simulink model "Final_Dual2"  (R2025a)
settings: Solver=ode113  StartTime=0.0  StopTime=1800  FixedStep=0.01  MaxStep=0.1  RelTol=1e-3
undefined symbols (not defined in the file or in its folder): sigbuilder_block
libraries: simulink x3784, slpidlib x2
(part 2 of 161)

== system Final_Dual2/VehicleDynamics//RoadLoadModel ==
  TqAct : Inport
  Veh_Mass : Inport  Port=2
  Road_mu : Inport  Port=3
  Gear_ratio : Inport  Port=4
  Tyre_radius : Inport  Port=5
  2 : Constant  Value=0  SampleTime=-1
  2pi : Constant  Value=2*pi  SampleTime=-1
  3 : Constant  Value=0  SampleTime=-1
  Add4 : Sum
  Constant : Constant
  Constant1 : Constant  Value=2*pi
  Constant2 : Constant  Value=60/1000
  Delay : Delay  DelayLength=1
  Divide{,1..3} (4 alike) : Product  Inputs=*/
  Gain1 : Gain  Gain=-1
  Integrator : Integrator
  Product{1..4} (4 alike) : Product
  Product5 : Product  Inputs=4
  Product9 : Product  Inputs=3
  Rate Transition : RateTransition
  Saturation : Saturate  UpperLimit=30000  LowerLimit=-30000
  Sec2Min : Gain  Gain=60
  Sum : Sum
  Switch1 : Switch  Criteria=u2 > Threshold  Threshold=10  SaturateOnIntegerOverflow=off  InputSameDT=off
  Switch2 : Switch  Criteria=u2 > Threshold  Threshold=-10  SaturateOnIntegerOverflow=off  InputSameDT=off
  TmEta : Gain  Gain=0.96
  g-value : Constant  Value=9.8  SampleTime=-1
  RPM : Outport
  tag scope: Vehicle_Acceleration=global, Vehicle_Speed_kmph=global, rpm_final=global
  wires:
  Road_mu/1 -> Product9/3
  Divide/1 -> Sum/2
  Product3/1 -> Divide1/2
  Tyre_radius/1 -> Product1/2, Product3/2, Divide/2
  Product4/1 -> Divide/1
  Divide2/1 -> [Vehicle_Acceleration], Integrator/1  "Vehicle acceleration"
  Sum/1 -> Divide2/1  "Traction Force"
  Integrator/1 -> Sec2Min/1  "velocity"
  2pi/1 -> Product3/1
  TqAct/1 -> TmEta/1
  Sec2Min/1 -> Divide1/1  "velocity in min"
  Divide1/1 -> Product2/1  "wheelrpm"
  Veh_Mass/1 -> Divide2/2, Product9/1
  g-value/1 -> Product9/2
  Product2/1 -> Saturation/1
  Switch1/1 -> Gain1/1
  2/1 -> Switch1/3
  Product9/1 -> Switch1/1, Switch2/3  "Friction loss"
  [rpm_final] -> Switch1/2, Switch2/2
  Switch2/1 -> Add4/2
  3/1 -> Switch2/1
  Gain1/1 -> Add4/1
  Add4/1 -> Sum/1
  Gear_ratio/1 -> Product4/2, Divide3/2, Product2/2
  TmEta/1 -> Product4/1
  Saturation/1 -> Delay/1, RPM/1  "Motor RPM"
  Delay/1 -> Rate Transition/1
  Rate Transition/1 -> Product5/1, [rpm_final]
  Constant/1 -> Divide3/1
  Constant1/1 -> Product1/1
  Divide3/1 -> Product5/2
  Product1/1 -> Product5/3
  Constant2/1 -> Product5/4
  Product5/1 -> [Vehicle_Speed_kmph]

== system Final_Dual2/WLTP (3) ==
  Demux : Demux  Tag=STV Demux  Outputs=1
      settings: DisplayOption=none
  FromWs : FromWorkspace  Tag=STV FromWs  VariableName=tuvar
      SigBuilderData=|
      | common.afterFinalStr = 'Extrapolate'
      | common.sampleTime = 0
      | dataSet.timeRange = [0 3593]
      | dataSet.name = 'Sheet1'
      | sbobj.Name = 'Signal Builder'
      | sbobj.Groups.Name = 'Sheet1'
      | sbobj.Groups.Signals.Name = 'WLTP'
      | sbobj.Groups.Signals.XData = [0 1 2 3 4 5 6 7 8 9 10 11 ... (3594 elements, 1x3594)]
      | sbobj.Groups.Signals.YData = [0 0 0 0 0 0 0 0 0 0 0 0.06 ... (3594 elements, 1x3594)]
      | sbobj.Groups.TimeRange = [0 3593]
  WLTP : Outport  Tag=STV Outport
  wires:
  Demux/1 -> WLTP/1
  FromWs/1 -> Demux/1

== system Final_Dual2/Battery1/Module1 ==
  Module_Current : Inport
  Add : Sum  Inputs=++++++++++
  Add1 : Sum  Inputs=++++++++++
  Constant : Constant  Value=10
  Divide : Product  Inputs=*/
  Scope : Scope
      settings: DataLoggingSaveFormat=Array
  Scope1 : Scope
      settings: DataLoggingVariableName=ScopeData3  DataLoggingSaveFormat=Array
  SubModule_1 : Subsystem
  SubModule_10 : Subsystem
  SubModule_2 : Subsystem
  SubModule_3 : Subsystem
  SubModule_4 : Subsystem
  SubModule_5 : Subsystem
  SubModule_6 : Subsystem
  SubModule_7 : Subsystem
  SubModule_8 : Subsystem
  SubModule_9 : Subsystem
  Module_Voltage : Outport
  Module_avg_Temp : Outport  Port=2
  wires:
  SubModule_4/2(SubModule_avg_temp) -> Add1/4
  Add/1 -> Module_Voltage/1, Scope/1
  [Module_Current] -> SubModule_5/1(Module_Current)
  [Module_Current] -> SubModule_9/1(Module_Current)
  [Module_Current] -> SubModule_2/1(Module_Current)
  [Module_Current] -> SubModule_3/1(Module_Current)
  [Module_Current] -> SubModule_7/1(Module_Current)
  Module_Current/1 -> [Module_Current]
  SubModule_1/1(SubModule_Voltage) -> Add/1
  [Module_Current] -> SubModule_1/1(Module_Current)
  [Module_Current] -> SubModule_4/1(Module_Current)
  SubModule_6/2(SubModule_avg_temp) -> Add1/6
  Divide/1 -> Module_avg_Temp/1, Scope1/1
  SubModule_5/1(SubModule_Voltage) -> Add/5
  [Module_Current] -> SubModule_8/1(Module_Current)
  SubModule_8/2(SubModule_avg_temp) -> Add1/8
  SubModule_5/2(SubModule_avg_temp) -> Add1/5
  SubModule_8/1(SubModule_Voltage) -> Add/8
  [Module_Current] -> SubModule_10/1(Module_Current)
  Constant/1 -> Divide/2
  SubModule_10/1(SubModule_Voltage) -> Add/10
  SubModule_10/2(SubModule_avg_temp) -> Add1/10
  SubModule_7/1(SubModule_Voltage) -> Add/7
  SubModule_9/2(SubModule_avg_temp) -> Add1/9
  SubModule_3/1(SubModule_Voltage) -> Add/3
  SubModule_4/1(SubModule_Voltage) -> Add/4
  SubModule_2/2(SubModule_avg_temp) -> Add1/2
  SubModule_3/2(SubModule_avg_temp) -> Add1/3
  SubModule_7/2(SubModule_avg_temp) -> Add1/7
  Add1/1 -> Divide/1
  SubModule_9/1(SubModule_Voltage) -> Add/9
  SubModule_6/1(SubModule_Voltage) -> Add/6
  SubModule_2/1(SubModule_Voltage) -> Add/2
  SubModule_1/2(SubModule_avg_temp) -> Add1/1
  [Module_Current] -> SubModule_6/1(Module_Current)

== system Final_Dual2/Battery1/Module2 ==
  Module_Current : Inport
  Add : Sum  Inputs=++++++++++
  Add1 : Sum  Inputs=++++++++++
  Constant : Constant  Value=10
  Divide : Product  Inputs=*/
  Scope : Scope
      settings: DataLoggingSaveFormat=Array
  Scope1 : Scope
      settings: DataLoggingVariableName=ScopeData3  DataLoggingSaveFormat=Array
  SubModule_1 : Subsystem
  SubModule_10 : Subsystem
  SubModule_2 : Subsystem
  SubModule_3 : Subsystem
  SubModule_4 : Subsystem
  SubModule_5 : Subsystem
  SubModule_6 : Subsystem
  SubModule_7 : Subsystem
  SubModule_8 : Subsystem
  SubModule_9 : Subsystem
  Module_Voltage : Outport
  Module_avg_Temp : Outport  Port=2
  wires:
  SubModule_4/2(SubModule_avg_temp) -> Add1/4
  Add/1 -> Module_Voltage/1, Scope/1
  [Module_Current] -> SubModule_5/1(Module_Current)
  [Module_Current] -> SubModule_9/1(Module_Current)
  [Module_Current] -> SubModule_2/1(Module_Current)
  [Module_Current] -> SubModule_3/1(Module_Current)
  [Module_Current] -> SubModule_7/1(Module_Current)
  Module_Current/1 -> [Module_Current]
  SubModule_1/1(SubModule_Voltage) -> Add/1
  [Module_Current] -> SubModule_1/1(Module_Current)
  [Module_Current] -> SubModule_4/1(Module_Current)
  SubModule_6/2(SubModule_avg_temp) -> Add1/6
  Divide/1 -> Module_avg_Temp/1, Scope1/1
  SubModule_5/1(SubModule_Voltage) -> Add/5
  [Module_Current] -> SubModule_8/1(Module_Current)
  SubModule_8/2(SubModule_avg_temp) -> Add1/8
  SubModule_5/2(SubModule_avg_temp) -> Add1/5
  SubModule_8/1(SubModule_Voltage) -> Add/8
  [Module_Current] -> SubModule_10/1(Module_Current)
  Constant/1 -> Divide/2
  SubModule_10/1(SubModule_Voltage) -> Add/10
  SubModule_10/2(SubModule_avg_temp) -> Add1/10
  SubModule_7/1(SubModule_Voltage) -> Add/7
  SubModule_9/2(SubModule_avg_temp) -> Add1/9
  SubModule_3/1(SubModule_Voltage) -> Add/3
  SubModule_4/1(SubModule_Voltage) -> Add/4
  SubModule_2/2(SubModule_avg_temp) -> Add1/2
  SubModule_3/2(SubModule_avg_temp) -> Add1/3
  SubModule_7/2(SubModule_avg_temp) -> Add1/7
  Add1/1 -> Divide/1
  SubModule_9/1(SubModule_Voltage) -> Add/9
  SubModule_6/1(SubModule_Voltage) -> Add/6
  SubModule_2/1(SubModule_Voltage) -> Add/2
  SubModule_1/2(SubModule_avg_temp) -> Add1/1
  [Module_Current] -> SubModule_6/1(Module_Current)

== system Final_Dual2/Battery1/Module3 ==
  Module_Current : Inport
  Add : Sum  Inputs=++++++++++
  Add1 : Sum  Inputs=++++++++++
  Constant : Constant  Value=10
  Divide : Product  Inputs=*/
  Scope : Scope
      settings: DataLoggingSaveFormat=Array
  Scope1 : Scope
      settings: DataLoggingVariableName=ScopeData3  DataLoggingSaveFormat=Array
  SubModule_1 : Subsystem
  SubModule_10 : Subsystem
  SubModule_2 : Subsystem
  SubModule_3 : Subsystem
  SubModule_4 : Subsystem
  SubModule_5 : Subsystem
  SubModule_6 : Subsystem
  SubModule_7 : Subsystem
  SubModule_8 : Subsystem
  SubModule_9 : Subsystem
  Module_Voltage : Outport
  Module_avg_Temp : Outport  Port=2
  wires:
  [Module_Current] -> SubModule_6/1(Module_Current)
  SubModule_1/2(SubModule_avg_temp) -> Add1/1
  SubModule_2/1(SubModule_Voltage) -> Add/2
  SubModule_6/1(SubModule_Voltage) -> Add/6
  SubModule_9/1(SubModule_Voltage) -> Add/9
  Add1/1 -> Divide/1
  SubModule_7/2(SubModule_avg_temp) -> Add1/7
  SubModule_3/2(SubModule_avg_temp) -> Add1/3
  SubModule_2/2(SubModule_avg_temp) -> Add1/2
  SubModule_4/1(SubModule_Voltage) -> Add/4
  SubModule_3/1(SubModule_Voltage) -> Add/3
  SubModule_9/2(SubModule_avg_temp) -> Add1/9
  SubModule_7/1(SubModule_Voltage) -> Add/7
  SubModule_10/2(SubModule_avg_temp) -> Add1/10
  SubModule_10/1(SubModule_Voltage) -> Add/10
  Constant/1 -> Divide/2
  [Module_Current] -> SubModule_10/1(Module_Current)
  SubModule_8/1(SubModule_Voltage) -> Add/8
  SubModule_5/2(SubModule_avg_temp) -> Add1/5
  SubModule_8/2(SubModule_avg_temp) -> Add1/8
  [Module_Current] -> SubModule_8/1(Module_Current)
  SubModule_5/1(SubModule_Voltage) -> Add/5
  Divide/1 -> Scope1/1, Module_avg_Temp/1
  SubModule_6/2(SubModule_avg_temp) -> Add1/6
  [Module_Current] -> SubModule_4/1(Module_Current)
  [Module_Current] -> SubModule_1/1(Module_Current)
  SubModule_1/1(SubModule_Voltage) -> Add/1
  Module_Current/1 -> [Module_Current]
  [Module_Current] -> SubModule_7/1(Module_Current)
  [Module_Current] -> SubModule_3/1(Module_Current)
  [Module_Current] -> SubModule_2/1(Module_Current)
  [Module_Current] -> SubModule_9/1(Module_Current)
  [Module_Current] -> SubModule_5/1(Module_Current)
  Add/1 -> Scope/1, Module_Voltage/1
  SubModule_4/2(SubModule_avg_temp) -> Add1/4

== system Final_Dual2/Battery1/NMC_Cell_Config ==
  A : Constant  Value=0.013
  C1_User1 : Constant  Value=[800 850 900 950 1000 1050 1000 950 900 850 800]
  C2_User : Constant  Value=[15 16 17 18 19 20 19 18 17 16 15]
  Cell_Capacity_Ah_rated : Constant  Value=26.5
  Gain1 : Gain  Gain=1e-03
  Gain2 : Gain
  Gain3 : Gain  Gain=1e-03
  Gain4 : Gain  Gain=1e+03
  Gain5 : Gain  Gain=0.01
  Gain6 : Gain  Gain=1e-04
  Goto11 : Goto  TagVisibility=global
  M*Cp : Constant  Value=369
  OCV_NMC : Constant  Value=|
      | [
      |     2.954364, 3.109857, 3.273534, 3.3066, 3.34,    3.3734,  3.20473;
      |     3.122427, 3.286765, 3.459753, 3.4947, 3.53,    3.5653,  3.387035;
      |     3.175499, 3.342631, 3.518559, 3.5541, 3.59,    3.6259,  3.444605;
      |     3.210881, 3.379875, 3.557763, 3.5937, 3.63,    3.6663,  3.482985;
      |     3.237417, 3.407808, 3.587166, 3.6234, 3.66,    3.6966,  3.511777;
      |     3.272799, 3.445052, 3.62637,  3.663,  3.7,     3.737,   3.55015;
      |     3.317026, 3.491066, 3.675375, 3.7125, 3.75,    3.7875,  3.598125;
      |     3.387789, 3.566094, 3.753783, 3.7917, 3.83,    3.8683,  3.674885;
      |     3.467398, 3.649892, 3.841992, 3.8808, 3.92,    3.9592,  3.76124;
      |     3.564697, 3.752313, 3.949803, 3.9897, 4.03,    4.0703,  3.866785;
      |     3.653151, 3.845422, 4.047813, 4.0887, 4.13,    4.1713,  3.962735
      | ]
  R1_User : Constant  Value=[1.5 1.2 0.9 0.7 0.6 0.5 0.5 0.5 0.6 0.7 0.8]
  R2_User1 : Constant  Value=[2.5 2 1.6 1.3 1.1 1 1.1 1.2 1.3 1.4 1.5]
  Ri_NMC : Constant  Value=|
      | [67.2155, 61.105, 55.55, 55, 52.25, 49.6375, 54.60125;
      |     48.884, 44.44, 40.4, 40, 38, 36.1, 39.71;
      |     44.60665, 40.5515, 36.865, 36.5, 34.675, 32.94125, 36.23538;
      |     41.5514, 37.774, 34.34, 34, 32.83, 30.685, 33.7535;
      |     40.3293, 36.663, 33.33, 33, 31.35, 29.7825, 32.76075;
      |     39.71825, 36.1075, 32.825, 32.5, 31.25, 29.33125, 32.26438;
      |     40.08488, 36.4408, 33.128, 32.8, 31.16, 29.602, 32.5622;
      |     40.94035, 37.2185, 33.835, 33.5, 31.825, 30.23375, 33.15738;
      |     42.7735, 38.1925, 35.03, 34.7, 32.375, 31.5875, 34.74263;
      |     51.3282, 46.602, 42.42, 42, 39.9, 37.905, 41.6955;
      |     73.326, 66.66, 60.6, 60, 57, 54.15, 59.565]
  SOC_Initial_% : Constant  Value=100
  SOC_User : Constant  Value=[0 10 20 30 40 50 60 70 80 90 100]
  Temp_Initial_degC : Constant  Value=25
  Temp_ambient : Constant  Value=25
  h : Constant  Value=20
  tag scope: C1_User=global, C2_User=global, Cell_Capacity=global, Cp=global, OCV=global, R1_User=global, R2_User=global, Ri_User=global, SOC_Iinitial=global, SOC_User=global, Temp_Iinitial=global, Temp_ambient=global, h=global
  wires:
  OCV_NMC/1 -> [OCV]
  SOC_User/1 -> Gain5/1
  R1_User/1 -> Gain1/1
  Gain1/1 -> [R1_User]
  C1_User1/1 -> Gain2/1
  Gain2/1 -> [C1_User]
  R2_User1/1 -> Gain3/1
  Gain3/1 -> [R2_User]
  Gain4/1 -> [C2_User]
  C2_User/1 -> Gain4/1
  Cell_Capacity_Ah_rated/1 -> [Cell_Capacity]
  SOC_Initial_%/1 -> [SOC_Iinitial]
  Gain5/1 -> [SOC_User]
  Temp_Initial_degC/1 -> [Temp_ambient], [Temp_Iinitial]
  h/1 -> [h]
  A/1 -> Goto11/1
  M*Cp/1 -> [Cp]
  Gain6/1 -> [Ri_User]
  Ri_NMC/1 -> Gain6/1

== system Final_Dual2/Battery1/SOCEstimator ==
  SOC_Initial : Inport
  Pack_Capacity : Inport  Port=2
  Current : Inport  Port=3
  SOCEstimator : Subsystem
  SOC : Outport
  wires:
  SOCEstimator/1(SOC) -> SOC/1
  SOC_Initial/1 -> SOCEstimator/1(SOC_Initial)
  Current/1 -> SOCEstimator/2(Current)
  Pack_Capacity/1 -> SOCEstimator/3(CellCapacity)

== system Final_Dual2/Battery2/LTO_Cell_Config ==
  A : Constant  Value=0.0344
  C1_User1 : Constant  Value=[5.0, 9.0, 12.0, 14.0, 14.8, 15.0, 14.8, 13.0, 10.0, 7.0, 4.5]
  C2_User : Constant  Value=[50, 90, 130, 160, 168, 170, 168, 155, 120, 80, 45]
  Cell_Capacity_Ah_rated : Constant  Value=23
  Gain1 : Gain  Gain=1e-03
  Gain2 : Gain  Gain=1e+03
  Gain3 : Gain  Gain=1e-03
  Gain4 : Gain  Gain=1e+03
  Gain5 : Gain  Gain=0.01
  Gain6 : Gain  Gain=1e-03
  M*Cp : Constant  Value=632.5
  OCV_LTO : Constant  Value=|
      | [1.79,  1.77,   1.76,   1.74,   1.71,   1.69,   1.66;
      |     2.09,  2.09,   2.08,   2.07,   2.06,   2.05,   2.04;
      |     2.19,  2.19,   2.18,   2.18,   2.17,   2.16,   2.15;
      |     2.23,  2.23,   2.23,   2.22,   2.22,   2.21,   2.21;
      |     2.25,  2.25,   2.25,   2.24,   2.24,   2.23,   2.23;
      |     2.28,  2.27,   2.27,   2.27,   2.26,   2.26,   2.25;
      |     2.30,  2.29,   2.29,   2.29,   2.28,   2.28,   2.27;
      |     2.32,  2.31,   2.31,   2.31,   2.30,   2.30,   2.29;
      |     2.34,  2.34,   2.34,   2.33,   2.33,   2.32,   2.31;
      |     2.39,  2.39,   2.38,   2.38,   2.37,   2.36,   2.35;
      |     2.64,  2.62,   2.61,   2.60,   2.59,   2.58,   2.57]
  R1_User : Constant  Value=[1.00, 0.65, 0.50, 0.40, 0.37, 0.35, 0.37, 0.45, 0.60, 0.80, 1.10]
  R2_User1 : Constant  Value=[2.00, 1.20, 0.90, 0.70, 0.62, 0.60, 0.62, 0.75, 1.00, 1.50, 2.20]
  Ri_LTO : Constant  Value=[2.50,1.90,1.65,1.50,1.40,1.30,1.25;1.50,1.10,0.90,0.80,0.75,0.72,0.70;1.25,0.95,0.75,0.65,0.60,0.58,0.57;1.10,0.80,0.60,0.52,0.48,0.47,0.46;1.05,0.75,0.55,0.48,0.45,0.44,0.43;1.00,0.70,0.52,0.45,0.42,0.41,0.40;1.05,0.75,0.55,0.48,0.45,0.44,0.43;1.15,0.85,0.65,0.57,0.53,0.51,0.50;1.40,1.05,0.85,0.75,0.70,0.68,0.67;1.80,1.40,1.15,1.00,0.90,0.85,0.82;2.20,1.70,1.40,1.25,1.15,1.10,1.05]
  SOC_Initial_% : Constant  Value=100
  SOC_User : Constant  Value=[0 10 20 30 40 50 60 70 80 90 100]
  Temp_Initial_degC : Constant  Value=25
  h : Constant  Value=25
  tag scope: A_LTO=global, C1_User_LTO=global, C2_User_LTO=global, Cell_Capacity_LTO=global, Cp_LTO=global, OCV_LTO=global, R1_User_LTO=global, R2_User_LTO=global, Ri_User_LTO=global, SOC_Iinitial_LTO=global, SOC_User_LTO=global, Temp_Iinitial_LTO=global, h_LTO=global
  wires:
  OCV_LTO/1 -> [OCV_LTO]
  SOC_User/1 -> Gain5/1
  R1_User/1 -> Gain1/1
  Gain1/1 -> [R1_User_LTO]
  C1_User1/1 -> Gain2/1
  Gain2/1 -> [C1_User_LTO]
  R2_User1/1 -> Gain3/1
  Gain3/1 -> [R2_User_LTO]
  Gain4/1 -> [C2_User_LTO]
  C2_User/1 -> Gain4/1
  Cell_Capacity_Ah_rated/1 -> [Cell_Capacity_LTO]
  SOC_Initial_%/1 -> [SOC_Iinitial_LTO]
  Gain5/1 -> [SOC_User_LTO]
  Temp_Initial_degC/1 -> [Temp_Iinitial_LTO]
  h/1 -> [h_LTO]
  A/1 -> [A_LTO]
  M*Cp/1 -> [Cp_LTO]
  Gain6/1 -> [Ri_User_LTO]
  Ri_LTO/1 -> Gain6/1

== system Final_Dual2/Battery2/Module1 ==
  Module_Current : Inport
  Add : Sum
  Add1 : Sum
  Constant : Constant  Value=2
  Divide : Product  Inputs=*/
  Scope : Scope
      settings: DataLoggingSaveFormat=Array
  Scope1 : Scope
      settings: ActiveDisplayYMinimum=53.8572  ActiveDisplayYMaximum=77.3331  DataLoggingVariableName=ScopeData3  DataLoggingSaveFormat=Array
  SubModule_1 : Subsystem
  SubModule_2 : Subsystem
  Module_Voltage : Outport
  Module_avg_Temp : Outport  Port=2
  wires:
  Add/1 -> Module_Voltage/1, Scope/1
  Module_Current/1 -> [Module_Current]
  SubModule_1/1(SubModule_Voltage) -> Add/1
  [Module_Current] -> SubModule_1/1(Module_Current)
  Divide/1 -> Module_avg_Temp/1, Scope1/1
  Constant/1 -> Divide/2
  Add1/1 -> Divide/1
  [Module_Current] -> SubModule_2/1(Module_Current)
  SubModule_2/1(SubModule_Voltage) -> Add/2
  SubModule_1/2(SubModule_avg_temp) -> Add1/1
  SubModule_2/2(SubModule_avg_temp) -> Add1/2

== system Final_Dual2/Battery2/Module2 ==
  Module_Current : Inport
  Add : Sum
  Add1 : Sum
  Constant : Constant  Value=2
  Divide : Product  Inputs=*/
  Scope : Scope
      settings: DataLoggingSaveFormat=Array
  Scope1 : Scope
      settings: ActiveDisplayYMinimum=53.8572  ActiveDisplayYMaximum=77.3331  DataLoggingVariableName=ScopeData3  DataLoggingSaveFormat=Array
  SubModule_1 : Subsystem
  SubModule_2 : Subsystem
  Module_Voltage : Outport
  Module_avg_Temp : Outport  Port=2
  wires:
  SubModule_2/2(SubModule_avg_temp) -> Add1/2
  SubModule_1/2(SubModule_avg_temp) -> Add1/1
  SubModule_2/1(SubModule_Voltage) -> Add/2
  [Module_Current] -> SubModule_2/1(Module_Current)
  Add1/1 -> Divide/1
  Constant/1 -> Divide/2
  Divide/1 -> Scope1/1, Module_avg_Temp/1
  [Module_Current] -> SubModule_1/1(Module_Current)
  SubModule_1/1(SubModule_Voltage) -> Add/1
  Module_Current/1 -> [Module_Current]
  Add/1 -> Scope/1, Module_Voltage/1

== system Final_Dual2/Battery2/SOCEstimator ==
  SOC_Initial : Inport
  Pack_Capacity : Inport  Port=2
  Current : Inport  Port=3
  SOCEstimator : Subsystem
  SOC : Outport
  wires:
  SOCEstimator/1(SOC) -> SOC/1
  SOC_Initial/1 -> SOCEstimator/1(SOC_Initial)
  Current/1 -> SOCEstimator/2(Current)
  Pack_Capacity/1 -> SOCEstimator/3(CellCapacity)

== system Final_Dual2/Observations/Battery1 Operation ==
  Battery1_Voltage : Inport
  Battery1_Current : Inport  Port=2
  Battery1_DischargeCurrLim : Inport  Port=3
  Battery1_ChargeCurrLim : Inport  Port=4
  Battery1_SOC : Inport  Port=5
  Battery1_Temperature : Inport  Port=6
  Battery1_Power : Inport  Port=7
  Battery1_Currents,Current_Limits&SOC : Scope  NumInputPorts=2
      settings: ActiveDisplayYMinimum=-203.9141  ActiveDisplayYMaximum=272.28558  DataLoggingVariableName=ScopeData2
  Battery1_Power&Temperature : Scope  NumInputPorts=2
      settings: ActiveDisplayYMinimum=24.76608  ActiveDisplayYMaximum=27.10528  DataLoggingVariableName=ScopeData3
  Battery1_Voltage&SOC : Scope  NumInputPorts=2
      settings: ActiveDisplayYMinimum=749.76765  ActiveDisplayYMaximum=933.2467
  Mux : Mux  Inputs=3
  wires:
  Battery1_Voltage/1 -> Battery1_Voltage&SOC/1
  Battery1_SOC/1 -> Battery1_Voltage&SOC/2, Battery1_Currents,Current_Limits&SOC/2
  Mux/1 -> Battery1_Currents,Current_Limits&SOC/1
  Battery1_Current/1 -> Mux/1
  Battery1_DischargeCurrLim/1 -> Mux/2
  Battery1_ChargeCurrLim/1 -> Mux/3
  Battery1_Temperature/1 -> Battery1_Power&Temperature/1
  Battery1_Power/1 -> Battery1_Power&Temperature/2

== system Final_Dual2/Observations/Battery2 Operation ==
  Battery2_Voltage : Inport
  Battery2_Current : Inport  Port=2
  Battery2_DischargeCurrLim : Inport  Port=3
  Battery2_ChargeCurrLim : Inport  Port=4
  Battery2_SOC : Inport  Port=5
  Battery2_Temperature : Inport  Port=6
  Battery2_Power : Inport  Port=7
  Battery2_Currents,Current_Limits&SOC : Scope  NumInputPorts=2
      settings: ActiveDisplayYMinimum=-965.27695  ActiveDisplayYMaximum=1034.84646  DataLoggingVariableName=ScopeData2
  Battery2_Power&Temperature : Scope  NumInputPorts=2
      settings: DataLoggingVariableName=ScopeData3
  Battery2_Voltage&SOC : Scope  NumInputPorts=2
      settings: ActiveDisplayYMinimum=63.66915  ActiveDisplayYMaximum=145.68331
  Mux : Mux  Inputs=3
  wires:
  Battery2_SOC/1 -> Battery2_Voltage&SOC/2, Battery2_Currents,Current_Limits&SOC/2
  Battery2_Voltage/1 -> Battery2_Voltage&SOC/1
  Battery2_ChargeCurrLim/1 -> Mux/3
  Battery2_Temperature/1 -> Battery2_Power&Temperature/1
  Battery2_Power/1 -> Battery2_Power&Temperature/2
  Battery2_DischargeCurrLim/1 -> Mux/2
  Battery2_Current/1 -> Mux/1
  Mux/1 -> Battery2_Currents,Current_Limits&SOC/1

== system Final_Dual2/Observations/DAB & Load Splitter Operation ==
  DAB_HighSideCurrentRef : Inport
  DAB_HighSideCurrent : Inport  Port=2
  DAB_PowerTransfer : Inport  Port=3
  Battery1_Current : Inport  Port=4
  Battery2_Current : Inport  Port=5
  Total_Current : Inport  Port=6
  Currents : Scope  NumInputPorts=2
      settings: ActiveDisplayYMinimum=-101.22034  ActiveDisplayYMaximum=330.24185  DataLoggingVariableName=ScopeData6
  DAB_HighSideCurr : Scope  NumInputPorts=2
      settings: ActiveDisplayYMinimum=-74.13996  ActiveDisplayYMaximum=160.56624  DataLoggingVariableName=ScopeData4
  DAB_Power : Scope
      settings: ActiveDisplayYMinimum=-56.99649  ActiveDisplayYMaximum=71.85076  DataLoggingVariableName=ScopeData5
  Mux : Mux  Inputs=3
  wires:
  DAB_PowerTransfer/1 -> DAB_Power/1
  DAB_HighSideCurrent/1 -> DAB_HighSideCurr/2, Mux/2
  Battery1_Current/1 -> Mux/1
  Total_Current/1 -> Mux/3
  DAB_HighSideCurrentRef/1 -> DAB_HighSideCurr/1
  Mux/1 -> Currents/1
  Battery2_Current/1 -> Currents/2

== system Final_Dual2/Observations/System Operation ==
  RPM_request : Inport
  RPM_Actual : Inport  Port=2
  Vehicle_Speed : Inport  Port=3
  Electrical_Power : Inport  Port=4
  Mechanical_Power : Inport  Port=5
  System_Efficiency : Inport  Port=6
  Driveline_Torque_Request : Inport  Port=7
  Driveline_Torque : Inport  Port=8
  Motor_Torque : Inport  Port=9
  Vehicle_Acceleration : Inport  Port=10
  Mux : Mux  Inputs=2
  Mux1 : Mux  Inputs=2
  Mux2 : Mux  Inputs=2
  Power&Efficiency : Scope  NumInputPorts=2
      settings: ActiveDisplayYMinimum=-94.56358  ActiveDisplayYMaximum=255.83618  DataLoggingVariableName=ScopeData8
  RPM_Requested&Actual : Scope  NumInputPorts=2
      settings: ActiveDisplayYMinimum=-2187.5  ActiveDisplayYMaximum=19687.5  DataLoggingVariableName=ScopeData7
  Requested&Actual_Torques : Scope  NumInputPorts=2
      settings: ActiveDisplayYMinimum=-861.66528  ActiveDisplayYMaximum=540.18503  DataLoggingVariableName=ScopeData9
  VehicleSpeed&Acceleration : Scope  NumInputPorts=2
      settings: ActiveDisplayYMinimum=-2187.5  ActiveDisplayYMaximum=19687.5  DataLoggingVariableName=ScopeData10
  wires:
  RPM_request/1 -> Mux2/1
  RPM_Actual/1 -> Mux2/2
  Electrical_Power/1 -> Mux/1
  Mechanical_Power/1 -> Mux/2
  System_Efficiency/1 -> Power&Efficiency/2
  Mux/1 -> Power&Efficiency/1
  Mux1/1 -> Requested&Actual_Torques/1
  Driveline_Torque_Request/1 -> Mux1/1
  Driveline_Torque/1 -> Mux1/2
  Motor_Torque/1 -> Requested&Actual_Torques/2
  Vehicle_Speed/1 -> VehicleSpeed&Acceleration/1, RPM_Requested&Actual/2
  Mux2/1 -> RPM_Requested&Actual/1
  Vehicle_Acceleration/1 -> VehicleSpeed&Acceleration/2

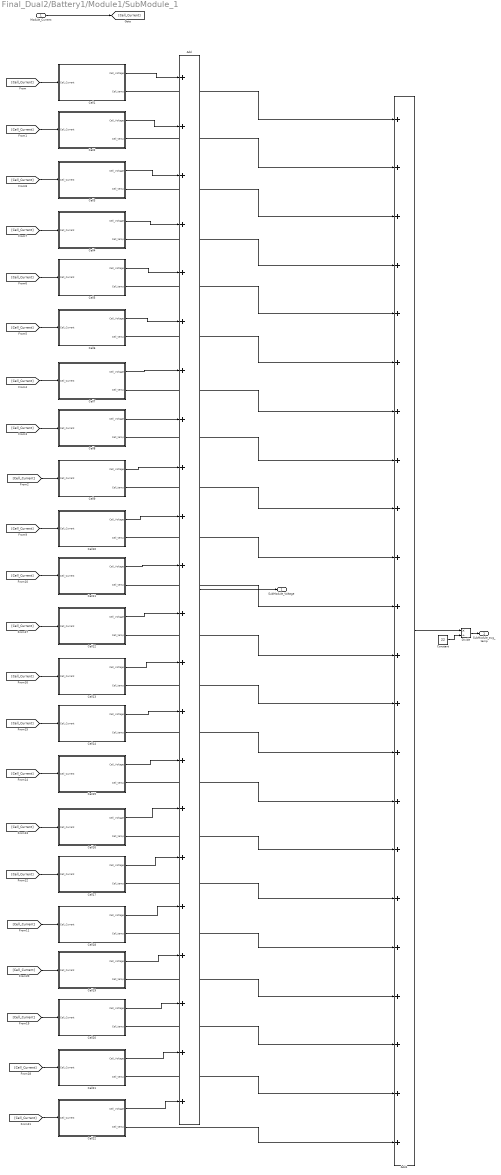
== system Final_Dual2/Battery1/Module1/SubModule_1 ==
  Module_Current : Inport
  Add : Sum  Inputs=++++++++++++++++++++++
  Add1 : Sum  Inputs=++++++++++++++++++++++
  Cell1 : Subsystem
  Cell10 : Subsystem
  Cell11 : Subsystem
  Cell12 : Subsystem
  Cell13 : Subsystem
  Cell14 : Subsystem
  Cell15 : Subsystem
  Cell16 : Subsystem
  Cell17 : Subsystem
  Cell18 : Subsystem
  Cell19 : Subsystem
  Cell2 : Subsystem
  Cell20 : Subsystem
  Cell21 : Subsystem
  Cell22 : Subsystem
  Cell3 : Subsystem
  Cell4 : Subsystem
  Cell5 : Subsystem
  Cell6 : Subsystem
  Cell7 : Subsystem
  Cell8 : Subsystem
  Cell9 : Subsystem
  Constant : Constant  Value=22
  Divide : Product  Inputs=*/
  SubModule_Voltage : Outport
  SubModule_avg_temp : Outport  Port=2
  wires:
  Cell9/2(Cell_temp) -> Add1/9
  [Cell_Current] -> Cell8/1(Cell_Current)
  Cell13/1(Cell_Voltage) -> Add/13
  Cell4/1(Cell_Voltage) -> Add/4
  Module_Current/1 -> [Cell_Current]
  Cell15/1(Cell_Voltage) -> Add/15
  [Cell_Current] -> Cell7/1(Cell_Current)
  [Cell_Current] -> Cell10/1(Cell_Current)
  Cell21/2(Cell_temp) -> Add1/21
  Cell5/1(Cell_Voltage) -> Add/5
  [Cell_Current] -> Cell1/1(Cell_Current)
  Cell2/1(Cell_Voltage) -> Add/2
  Cell19/1(Cell_Voltage) -> Add/19
  [Cell_Current] -> Cell5/1(Cell_Current)
  [Cell_Current] -> Cell11/1(Cell_Current)
  Cell6/1(Cell_Voltage) -> Add/6
  Cell11/1(Cell_Voltage) -> Add/11
  [Cell_Current] -> Cell18/1(Cell_Current)
  Cell7/2(Cell_temp) -> Add1/7
  [Cell_Current] -> Cell21/1(Cell_Current)
  [Cell_Current] -> Cell12/1(Cell_Current)
  [Cell_Current] -> Cell4/1(Cell_Current)
  Cell18/1(Cell_Voltage) -> Add/18
  Cell20/1(Cell_Voltage) -> Add/20
  Cell11/2(Cell_temp) -> Add1/11
  [Cell_Current] -> Cell2/1(Cell_Current)
  Cell16/2(Cell_temp) -> Add1/16
  [Cell_Current] -> Cell15/1(Cell_Current)
  [Cell_Current] -> Cell6/1(Cell_Current)
  [Cell_Current] -> Cell13/1(Cell_Current)
  Cell2/2(Cell_temp) -> Add1/2
  Cell22/2(Cell_temp) -> Add1/22
  Cell9/1(Cell_Voltage) -> Add/9
  Cell7/1(Cell_Voltage) -> Add/7
  [Cell_Current] -> Cell9/1(Cell_Current)
  Cell14/2(Cell_temp) -> Add1/14
  Cell17/1(Cell_Voltage) -> Add/17
  Cell10/2(Cell_temp) -> Add1/10
  [Cell_Current] -> Cell16/1(Cell_Current)
  Cell8/1(Cell_Voltage) -> Add/8
  Cell21/1(Cell_Voltage) -> Add/21
  Cell12/2(Cell_temp) -> Add1/12
  Cell22/1(Cell_Voltage) -> Add/22
  [Cell_Current] -> Cell20/1(Cell_Current)
  [Cell_Current] -> Cell17/1(Cell_Current)
  Cell10/1(Cell_Voltage) -> Add/10
  Cell18/2(Cell_temp) -> Add1/18
  Cell14/1(Cell_Voltage) -> Add/14
  Cell16/1(Cell_Voltage) -> Add/16
  [Cell_Current] -> Cell3/1(Cell_Current)
  Cell12/1(Cell_Voltage) -> Add/12
  Cell20/2(Cell_temp) -> Add1/20
  Cell1/1(Cell_Voltage) -> Add/1
  [Cell_Current] -> Cell19/1(Cell_Current)
  Cell3/1(Cell_Voltage) -> Add/3
  [Cell_Current] -> Cell22/1(Cell_Current)
  [Cell_Current] -> Cell14/1(Cell_Current)
  Cell19/2(Cell_temp) -> Add1/19
  Cell6/2(Cell_temp) -> Add1/6
  Cell17/2(Cell_temp) -> Add1/17
  Cell15/2(Cell_temp) -> Add1/15
  Cell8/2(Cell_temp) -> Add1/8
  Cell3/2(Cell_temp) -> Add1/3
  Cell13/2(Cell_temp) -> Add1/13
  Add/1 -> SubModule_Voltage/1
  Cell4/2(Cell_temp) -> Add1/4
  Cell5/2(Cell_temp) -> Add1/5
  Cell1/2(Cell_temp) -> Add1/1
  Add1/1 -> Divide/1
  Constant/1 -> Divide/2
  Divide/1 -> SubModule_avg_temp/1

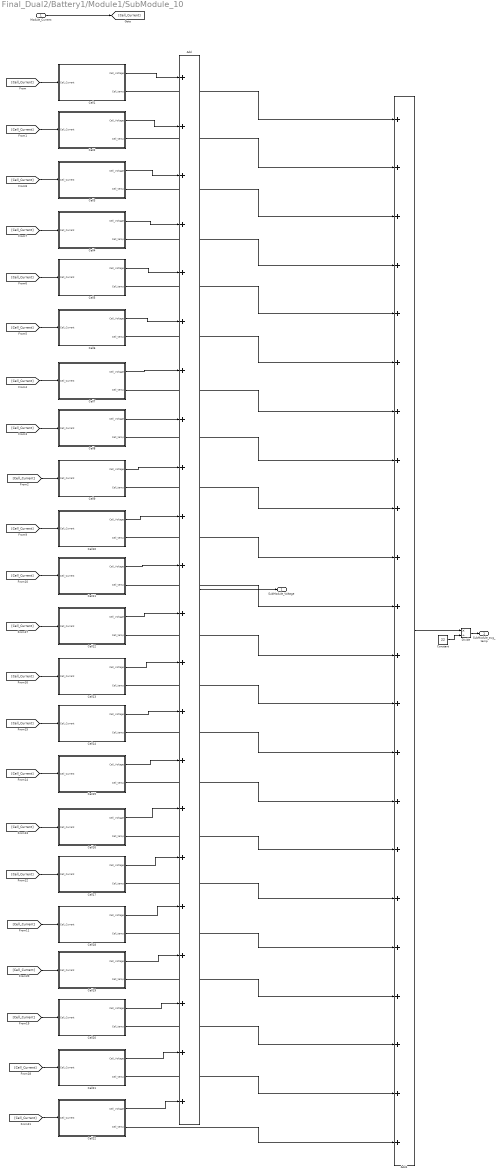
== system Final_Dual2/Battery1/Module1/SubModule_10 ==
  Module_Current : Inport
  Add : Sum  Inputs=++++++++++++++++++++++
  Add1 : Sum  Inputs=++++++++++++++++++++++
  Cell1 : Subsystem
  Cell10 : Subsystem
  Cell11 : Subsystem
  Cell12 : Subsystem
  Cell13 : Subsystem
  Cell14 : Subsystem
  Cell15 : Subsystem
  Cell16 : Subsystem
  Cell17 : Subsystem
  Cell18 : Subsystem
  Cell19 : Subsystem
  Cell2 : Subsystem
  Cell20 : Subsystem
  Cell21 : Subsystem
  Cell22 : Subsystem
  Cell3 : Subsystem
  Cell4 : Subsystem
  Cell5 : Subsystem
  Cell6 : Subsystem
  Cell7 : Subsystem
  Cell8 : Subsystem
  Cell9 : Subsystem
  Constant : Constant  Value=22
  Divide : Product  Inputs=*/
  SubModule_Voltage : Outport
  SubModule_avg_temp : Outport  Port=2
  wires:
  Cell9/2(Cell_temp) -> Add1/9
  [Cell_Current] -> Cell8/1(Cell_Current)
  Cell13/1(Cell_Voltage) -> Add/13
  Cell4/1(Cell_Voltage) -> Add/4
  Module_Current/1 -> [Cell_Current]
  Cell15/1(Cell_Voltage) -> Add/15
  [Cell_Current] -> Cell7/1(Cell_Current)
  [Cell_Current] -> Cell10/1(Cell_Current)
  Cell21/2(Cell_temp) -> Add1/21
  Cell5/1(Cell_Voltage) -> Add/5
  [Cell_Current] -> Cell1/1(Cell_Current)
  Cell2/1(Cell_Voltage) -> Add/2
  Cell19/1(Cell_Voltage) -> Add/19
  [Cell_Current] -> Cell5/1(Cell_Current)
  [Cell_Current] -> Cell11/1(Cell_Current)
  Cell6/1(Cell_Voltage) -> Add/6
  Cell11/1(Cell_Voltage) -> Add/11
  [Cell_Current] -> Cell18/1(Cell_Current)
  Cell7/2(Cell_temp) -> Add1/7
  [Cell_Current] -> Cell21/1(Cell_Current)
  [Cell_Current] -> Cell12/1(Cell_Current)
  [Cell_Current] -> Cell4/1(Cell_Current)
  Cell18/1(Cell_Voltage) -> Add/18
  Cell20/1(Cell_Voltage) -> Add/20
  Cell11/2(Cell_temp) -> Add1/11
  [Cell_Current] -> Cell2/1(Cell_Current)
  Cell16/2(Cell_temp) -> Add1/16
  [Cell_Current] -> Cell15/1(Cell_Current)
  [Cell_Current] -> Cell6/1(Cell_Current)
  [Cell_Current] -> Cell13/1(Cell_Current)
  Cell2/2(Cell_temp) -> Add1/2
  Cell22/2(Cell_temp) -> Add1/22
  Cell9/1(Cell_Voltage) -> Add/9
  Cell7/1(Cell_Voltage) -> Add/7
  [Cell_Current] -> Cell9/1(Cell_Current)
  Cell14/2(Cell_temp) -> Add1/14
  Cell17/1(Cell_Voltage) -> Add/17
  Cell10/2(Cell_temp) -> Add1/10
  [Cell_Current] -> Cell16/1(Cell_Current)
  Cell8/1(Cell_Voltage) -> Add/8
  Cell21/1(Cell_Voltage) -> Add/21
  Cell12/2(Cell_temp) -> Add1/12
  Cell22/1(Cell_Voltage) -> Add/22
  [Cell_Current] -> Cell20/1(Cell_Current)
  [Cell_Current] -> Cell17/1(Cell_Current)
  Cell10/1(Cell_Voltage) -> Add/10
  Cell18/2(Cell_temp) -> Add1/18
  Cell14/1(Cell_Voltage) -> Add/14
  Cell16/1(Cell_Voltage) -> Add/16
  [Cell_Current] -> Cell3/1(Cell_Current)
  Cell12/1(Cell_Voltage) -> Add/12
  Cell20/2(Cell_temp) -> Add1/20
  Cell1/1(Cell_Voltage) -> Add/1
  [Cell_Current] -> Cell19/1(Cell_Current)
  Cell3/1(Cell_Voltage) -> Add/3
  [Cell_Current] -> Cell22/1(Cell_Current)
  [Cell_Current] -> Cell14/1(Cell_Current)
  Cell19/2(Cell_temp) -> Add1/19
  Cell6/2(Cell_temp) -> Add1/6
  Cell17/2(Cell_temp) -> Add1/17
  Cell15/2(Cell_temp) -> Add1/15
  Cell8/2(Cell_temp) -> Add1/8
  Cell3/2(Cell_temp) -> Add1/3
  Cell13/2(Cell_temp) -> Add1/13
  Add/1 -> SubModule_Voltage/1
  Cell4/2(Cell_temp) -> Add1/4
  Cell5/2(Cell_temp) -> Add1/5
  Cell1/2(Cell_temp) -> Add1/1
  Add1/1 -> Divide/1
  Constant/1 -> Divide/2
  Divide/1 -> SubModule_avg_temp/1

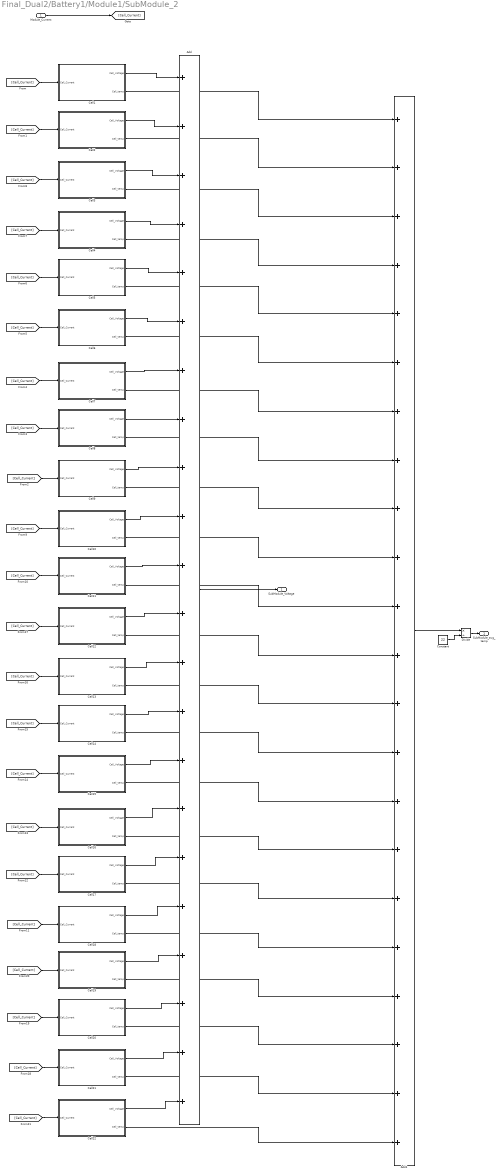
== system Final_Dual2/Battery1/Module1/SubModule_2 ==
  Module_Current : Inport
  Add : Sum  Inputs=++++++++++++++++++++++
  Add1 : Sum  Inputs=++++++++++++++++++++++
  Cell1 : Subsystem
  Cell10 : Subsystem
  Cell11 : Subsystem
  Cell12 : Subsystem
  Cell13 : Subsystem
  Cell14 : Subsystem
  Cell15 : Subsystem
  Cell16 : Subsystem
  Cell17 : Subsystem
  Cell18 : Subsystem
  Cell19 : Subsystem
  Cell2 : Subsystem
  Cell20 : Subsystem
  Cell21 : Subsystem
  Cell22 : Subsystem
  Cell3 : Subsystem
  Cell4 : Subsystem
  Cell5 : Subsystem
  Cell6 : Subsystem
  Cell7 : Subsystem
  Cell8 : Subsystem
  Cell9 : Subsystem
  Constant : Constant  Value=22
  Divide : Product  Inputs=*/
  SubModule_Voltage : Outport
  SubModule_avg_temp : Outport  Port=2
  wires:
  Divide/1 -> SubModule_avg_temp/1
  Constant/1 -> Divide/2
  Add1/1 -> Divide/1
  Cell1/2(Cell_temp) -> Add1/1
  Cell5/2(Cell_temp) -> Add1/5
  Cell4/2(Cell_temp) -> Add1/4
  Add/1 -> SubModule_Voltage/1
  Cell13/2(Cell_temp) -> Add1/13
  Cell3/2(Cell_temp) -> Add1/3
  Cell8/2(Cell_temp) -> Add1/8
  Cell15/2(Cell_temp) -> Add1/15
  Cell17/2(Cell_temp) -> Add1/17
  Cell6/2(Cell_temp) -> Add1/6
  Cell19/2(Cell_temp) -> Add1/19
  [Cell_Current] -> Cell14/1(Cell_Current)
  [Cell_Current] -> Cell22/1(Cell_Current)
  Cell3/1(Cell_Voltage) -> Add/3
  [Cell_Current] -> Cell19/1(Cell_Current)
  Cell1/1(Cell_Voltage) -> Add/1
  Cell20/2(Cell_temp) -> Add1/20
  Cell12/1(Cell_Voltage) -> Add/12
  [Cell_Current] -> Cell3/1(Cell_Current)
  Cell16/1(Cell_Voltage) -> Add/16
  Cell14/1(Cell_Voltage) -> Add/14
  Cell18/2(Cell_temp) -> Add1/18
  Cell10/1(Cell_Voltage) -> Add/10
  [Cell_Current] -> Cell17/1(Cell_Current)
  [Cell_Current] -> Cell20/1(Cell_Current)
  Cell22/1(Cell_Voltage) -> Add/22
  Cell12/2(Cell_temp) -> Add1/12
  Cell21/1(Cell_Voltage) -> Add/21
  Cell8/1(Cell_Voltage) -> Add/8
  [Cell_Current] -> Cell16/1(Cell_Current)
  Cell10/2(Cell_temp) -> Add1/10
  Cell17/1(Cell_Voltage) -> Add/17
  Cell14/2(Cell_temp) -> Add1/14
  [Cell_Current] -> Cell9/1(Cell_Current)
  Cell7/1(Cell_Voltage) -> Add/7
  Cell9/1(Cell_Voltage) -> Add/9
  Cell22/2(Cell_temp) -> Add1/22
  Cell2/2(Cell_temp) -> Add1/2
  [Cell_Current] -> Cell13/1(Cell_Current)
  [Cell_Current] -> Cell6/1(Cell_Current)
  [Cell_Current] -> Cell15/1(Cell_Current)
  Cell16/2(Cell_temp) -> Add1/16
  [Cell_Current] -> Cell2/1(Cell_Current)
  Cell11/2(Cell_temp) -> Add1/11
  Cell20/1(Cell_Voltage) -> Add/20
  Cell18/1(Cell_Voltage) -> Add/18
  [Cell_Current] -> Cell4/1(Cell_Current)
  [Cell_Current] -> Cell12/1(Cell_Current)
  [Cell_Current] -> Cell21/1(Cell_Current)
  Cell7/2(Cell_temp) -> Add1/7
  [Cell_Current] -> Cell18/1(Cell_Current)
  Cell11/1(Cell_Voltage) -> Add/11
  Cell6/1(Cell_Voltage) -> Add/6
  [Cell_Current] -> Cell11/1(Cell_Current)
  [Cell_Current] -> Cell5/1(Cell_Current)
  Cell19/1(Cell_Voltage) -> Add/19
  Cell2/1(Cell_Voltage) -> Add/2
  [Cell_Current] -> Cell1/1(Cell_Current)
  Cell5/1(Cell_Voltage) -> Add/5
  Cell21/2(Cell_temp) -> Add1/21
  [Cell_Current] -> Cell10/1(Cell_Current)
  [Cell_Current] -> Cell7/1(Cell_Current)
  Cell15/1(Cell_Voltage) -> Add/15
  Module_Current/1 -> [Cell_Current]
  Cell4/1(Cell_Voltage) -> Add/4
  Cell13/1(Cell_Voltage) -> Add/13
  [Cell_Current] -> Cell8/1(Cell_Current)
  Cell9/2(Cell_temp) -> Add1/9

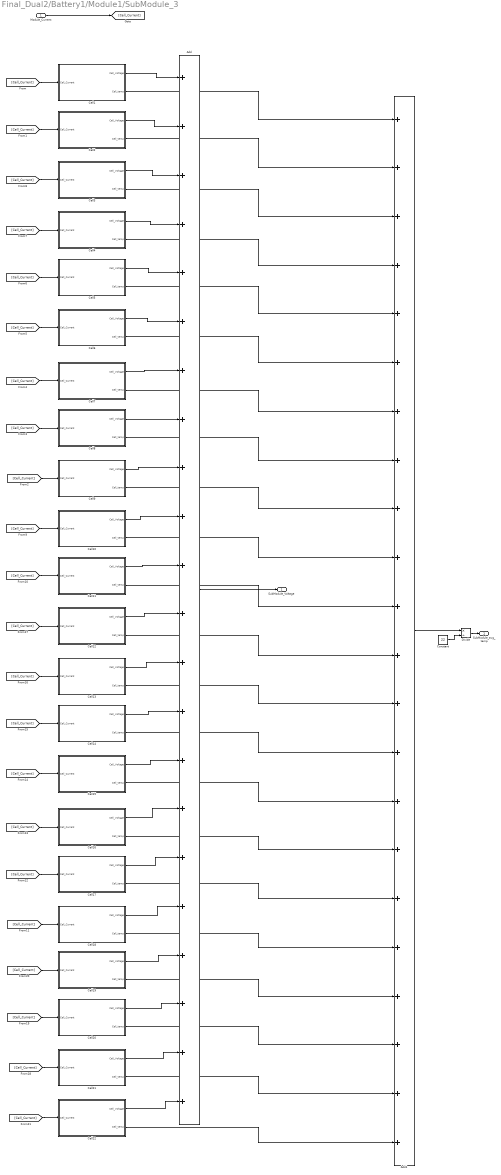
== system Final_Dual2/Battery1/Module1/SubModule_3 ==
  Module_Current : Inport
  Add : Sum  Inputs=++++++++++++++++++++++
  Add1 : Sum  Inputs=++++++++++++++++++++++
  Cell1 : Subsystem
  Cell10 : Subsystem
  Cell11 : Subsystem
  Cell12 : Subsystem
  Cell13 : Subsystem
  Cell14 : Subsystem
  Cell15 : Subsystem
  Cell16 : Subsystem
  Cell17 : Subsystem
  Cell18 : Subsystem
  Cell19 : Subsystem
  Cell2 : Subsystem
  Cell20 : Subsystem
  Cell21 : Subsystem
  Cell22 : Subsystem
  Cell3 : Subsystem
  Cell4 : Subsystem
  Cell5 : Subsystem
  Cell6 : Subsystem
  Cell7 : Subsystem
  Cell8 : Subsystem
  Cell9 : Subsystem
  Constant : Constant  Value=22
  Divide : Product  Inputs=*/
  SubModule_Voltage : Outport
  SubModule_avg_temp : Outport  Port=2
  wires:
  Cell9/2(Cell_temp) -> Add1/9
  [Cell_Current] -> Cell8/1(Cell_Current)
  Cell13/1(Cell_Voltage) -> Add/13
  Cell4/1(Cell_Voltage) -> Add/4
  Module_Current/1 -> [Cell_Current]
  Cell15/1(Cell_Voltage) -> Add/15
  [Cell_Current] -> Cell7/1(Cell_Current)
  [Cell_Current] -> Cell10/1(Cell_Current)
  Cell21/2(Cell_temp) -> Add1/21
  Cell5/1(Cell_Voltage) -> Add/5
  [Cell_Current] -> Cell1/1(Cell_Current)
  Cell2/1(Cell_Voltage) -> Add/2
  Cell19/1(Cell_Voltage) -> Add/19
  [Cell_Current] -> Cell5/1(Cell_Current)
  [Cell_Current] -> Cell11/1(Cell_Current)
  Cell6/1(Cell_Voltage) -> Add/6
  Cell11/1(Cell_Voltage) -> Add/11
  [Cell_Current] -> Cell18/1(Cell_Current)
  Cell7/2(Cell_temp) -> Add1/7
  [Cell_Current] -> Cell21/1(Cell_Current)
  [Cell_Current] -> Cell12/1(Cell_Current)
  [Cell_Current] -> Cell4/1(Cell_Current)
  Cell18/1(Cell_Voltage) -> Add/18
  Cell20/1(Cell_Voltage) -> Add/20
  Cell11/2(Cell_temp) -> Add1/11
  [Cell_Current] -> Cell2/1(Cell_Current)
  Cell16/2(Cell_temp) -> Add1/16
  [Cell_Current] -> Cell15/1(Cell_Current)
  [Cell_Current] -> Cell6/1(Cell_Current)
  [Cell_Current] -> Cell13/1(Cell_Current)
  Cell2/2(Cell_temp) -> Add1/2
  Cell22/2(Cell_temp) -> Add1/22
  Cell9/1(Cell_Voltage) -> Add/9
  Cell7/1(Cell_Voltage) -> Add/7
  [Cell_Current] -> Cell9/1(Cell_Current)
  Cell14/2(Cell_temp) -> Add1/14
  Cell17/1(Cell_Voltage) -> Add/17
  Cell10/2(Cell_temp) -> Add1/10
  [Cell_Current] -> Cell16/1(Cell_Current)
  Cell8/1(Cell_Voltage) -> Add/8
  Cell21/1(Cell_Voltage) -> Add/21
  Cell12/2(Cell_temp) -> Add1/12
  Cell22/1(Cell_Voltage) -> Add/22
  [Cell_Current] -> Cell20/1(Cell_Current)
  [Cell_Current] -> Cell17/1(Cell_Current)
  Cell10/1(Cell_Voltage) -> Add/10
  Cell18/2(Cell_temp) -> Add1/18
  Cell14/1(Cell_Voltage) -> Add/14
  Cell16/1(Cell_Voltage) -> Add/16
  [Cell_Current] -> Cell3/1(Cell_Current)
  Cell12/1(Cell_Voltage) -> Add/12
  Cell20/2(Cell_temp) -> Add1/20
  Cell1/1(Cell_Voltage) -> Add/1
  [Cell_Current] -> Cell19/1(Cell_Current)
  Cell3/1(Cell_Voltage) -> Add/3
  [Cell_Current] -> Cell22/1(Cell_Current)
  [Cell_Current] -> Cell14/1(Cell_Current)
  Cell19/2(Cell_temp) -> Add1/19
  Cell6/2(Cell_temp) -> Add1/6
  Cell17/2(Cell_temp) -> Add1/17
  Cell15/2(Cell_temp) -> Add1/15
  Cell8/2(Cell_temp) -> Add1/8
  Cell3/2(Cell_temp) -> Add1/3
  Cell13/2(Cell_temp) -> Add1/13
  Add/1 -> SubModule_Voltage/1
  Cell4/2(Cell_temp) -> Add1/4
  Cell5/2(Cell_temp) -> Add1/5
  Cell1/2(Cell_temp) -> Add1/1
  Add1/1 -> Divide/1
  Constant/1 -> Divide/2
  Divide/1 -> SubModule_avg_temp/1

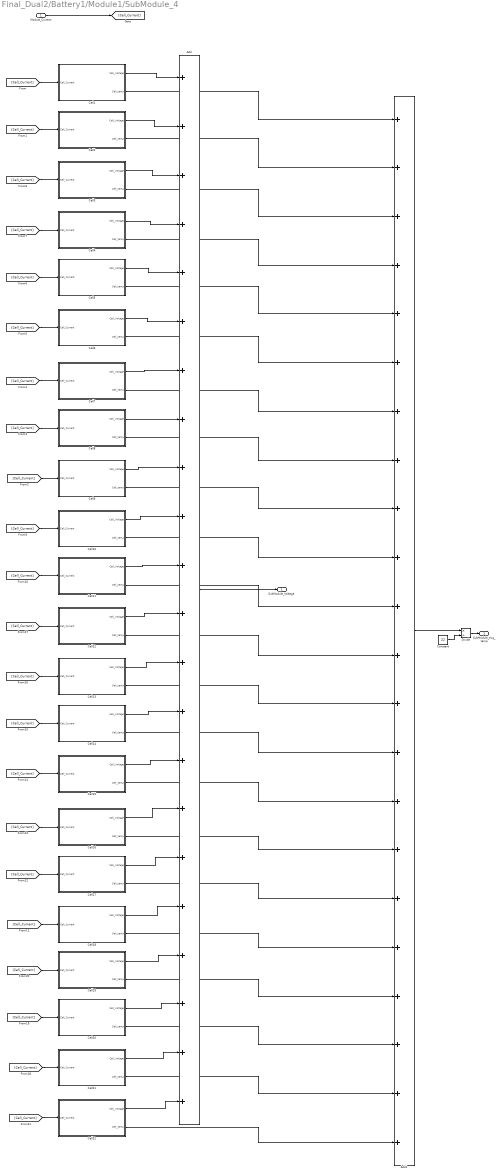
== system Final_Dual2/Battery1/Module1/SubModule_4 ==
  Module_Current : Inport
  Add : Sum  Inputs=++++++++++++++++++++++
  Add1 : Sum  Inputs=++++++++++++++++++++++
  Cell1 : Subsystem
  Cell10 : Subsystem
  Cell11 : Subsystem
  Cell12 : Subsystem
  Cell13 : Subsystem
  Cell14 : Subsystem
  Cell15 : Subsystem
  Cell16 : Subsystem
  Cell17 : Subsystem
  Cell18 : Subsystem
  Cell19 : Subsystem
  Cell2 : Subsystem
  Cell20 : Subsystem
  Cell21 : Subsystem
  Cell22 : Subsystem
  Cell3 : Subsystem
  Cell4 : Subsystem
  Cell5 : Subsystem
  Cell6 : Subsystem
  Cell7 : Subsystem
  Cell8 : Subsystem
  Cell9 : Subsystem
  Constant : Constant  Value=22
  Divide : Product  Inputs=*/
  SubModule_Voltage : Outport
  SubModule_avg_temp : Outport  Port=2
  wires:
  Divide/1 -> SubModule_avg_temp/1
  Constant/1 -> Divide/2
  Add1/1 -> Divide/1
  Cell1/2(Cell_temp) -> Add1/1
  Cell5/2(Cell_temp) -> Add1/5
  Cell4/2(Cell_temp) -> Add1/4
  Add/1 -> SubModule_Voltage/1
  Cell13/2(Cell_temp) -> Add1/13
  Cell3/2(Cell_temp) -> Add1/3
  Cell8/2(Cell_temp) -> Add1/8
  Cell15/2(Cell_temp) -> Add1/15
  Cell17/2(Cell_temp) -> Add1/17
  Cell6/2(Cell_temp) -> Add1/6
  Cell19/2(Cell_temp) -> Add1/19
  [Cell_Current] -> Cell14/1(Cell_Current)
  [Cell_Current] -> Cell22/1(Cell_Current)
  Cell3/1(Cell_Voltage) -> Add/3
  [Cell_Current] -> Cell19/1(Cell_Current)
  Cell1/1(Cell_Voltage) -> Add/1
  Cell20/2(Cell_temp) -> Add1/20
  Cell12/1(Cell_Voltage) -> Add/12
  [Cell_Current] -> Cell3/1(Cell_Current)
  Cell16/1(Cell_Voltage) -> Add/16
  Cell14/1(Cell_Voltage) -> Add/14
  Cell18/2(Cell_temp) -> Add1/18
  Cell10/1(Cell_Voltage) -> Add/10
  [Cell_Current] -> Cell17/1(Cell_Current)
  [Cell_Current] -> Cell20/1(Cell_Current)
  Cell22/1(Cell_Voltage) -> Add/22
  Cell12/2(Cell_temp) -> Add1/12
  Cell21/1(Cell_Voltage) -> Add/21
  Cell8/1(Cell_Voltage) -> Add/8
  [Cell_Current] -> Cell16/1(Cell_Current)
  Cell10/2(Cell_temp) -> Add1/10
  Cell17/1(Cell_Voltage) -> Add/17
  Cell14/2(Cell_temp) -> Add1/14
  [Cell_Current] -> Cell9/1(Cell_Current)
  Cell7/1(Cell_Voltage) -> Add/7
  Cell9/1(Cell_Voltage) -> Add/9
  Cell22/2(Cell_temp) -> Add1/22
  Cell2/2(Cell_temp) -> Add1/2
  [Cell_Current] -> Cell13/1(Cell_Current)
  [Cell_Current] -> Cell6/1(Cell_Current)
  [Cell_Current] -> Cell15/1(Cell_Current)
  Cell16/2(Cell_temp) -> Add1/16
  [Cell_Current] -> Cell2/1(Cell_Current)
  Cell11/2(Cell_temp) -> Add1/11
  Cell20/1(Cell_Voltage) -> Add/20
  Cell18/1(Cell_Voltage) -> Add/18
  [Cell_Current] -> Cell4/1(Cell_Current)
  [Cell_Current] -> Cell12/1(Cell_Current)
  [Cell_Current] -> Cell21/1(Cell_Current)
  Cell7/2(Cell_temp) -> Add1/7
  [Cell_Current] -> Cell18/1(Cell_Current)
  Cell11/1(Cell_Voltage) -> Add/11
  Cell6/1(Cell_Voltage) -> Add/6
  [Cell_Current] -> Cell11/1(Cell_Current)
  [Cell_Current] -> Cell5/1(Cell_Current)
  Cell19/1(Cell_Voltage) -> Add/19
  Cell2/1(Cell_Voltage) -> Add/2
  [Cell_Current] -> Cell1/1(Cell_Current)
  Cell5/1(Cell_Voltage) -> Add/5
  Cell21/2(Cell_temp) -> Add1/21
  [Cell_Current] -> Cell10/1(Cell_Current)
  [Cell_Current] -> Cell7/1(Cell_Current)
  Cell15/1(Cell_Voltage) -> Add/15
  Module_Current/1 -> [Cell_Current]
  Cell4/1(Cell_Voltage) -> Add/4
  Cell13/1(Cell_Voltage) -> Add/13
  [Cell_Current] -> Cell8/1(Cell_Current)
  Cell9/2(Cell_temp) -> Add1/9

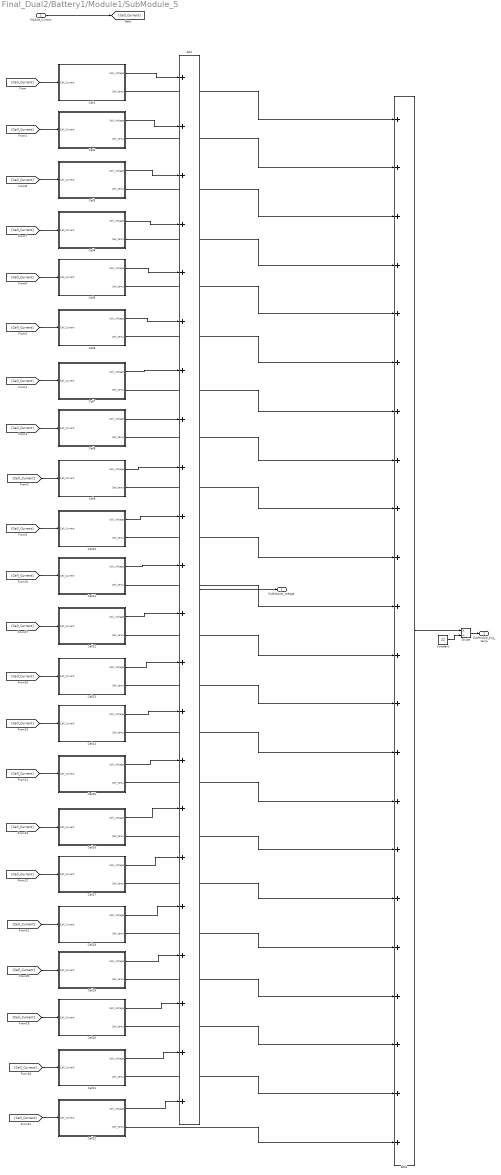
== system Final_Dual2/Battery1/Module1/SubModule_5 ==
  Module_Current : Inport
  Add : Sum  Inputs=++++++++++++++++++++++
  Add1 : Sum  Inputs=++++++++++++++++++++++
  Cell1 : Subsystem
  Cell10 : Subsystem
  Cell11 : Subsystem
  Cell12 : Subsystem
  Cell13 : Subsystem
  Cell14 : Subsystem
  Cell15 : Subsystem
  Cell16 : Subsystem
  Cell17 : Subsystem
  Cell18 : Subsystem
  Cell19 : Subsystem
  Cell2 : Subsystem
  Cell20 : Subsystem
  Cell21 : Subsystem
  Cell22 : Subsystem
  Cell3 : Subsystem
  Cell4 : Subsystem
  Cell5 : Subsystem
  Cell6 : Subsystem
  Cell7 : Subsystem
  Cell8 : Subsystem
  Cell9 : Subsystem
  Constant : Constant  Value=22
  Divide : Product  Inputs=*/
  SubModule_Voltage : Outport
  SubModule_avg_temp : Outport  Port=2
  wires:
  Cell9/2(Cell_temp) -> Add1/9
  [Cell_Current] -> Cell8/1(Cell_Current)
  Cell13/1(Cell_Voltage) -> Add/13
  Cell4/1(Cell_Voltage) -> Add/4
  Module_Current/1 -> [Cell_Current]
  Cell15/1(Cell_Voltage) -> Add/15
  [Cell_Current] -> Cell7/1(Cell_Current)
  [Cell_Current] -> Cell10/1(Cell_Current)
  Cell21/2(Cell_temp) -> Add1/21
  Cell5/1(Cell_Voltage) -> Add/5
  [Cell_Current] -> Cell1/1(Cell_Current)
  Cell2/1(Cell_Voltage) -> Add/2
  Cell19/1(Cell_Voltage) -> Add/19
  [Cell_Current] -> Cell5/1(Cell_Current)
  [Cell_Current] -> Cell11/1(Cell_Current)
  Cell6/1(Cell_Voltage) -> Add/6
  Cell11/1(Cell_Voltage) -> Add/11
  [Cell_Current] -> Cell18/1(Cell_Current)
  Cell7/2(Cell_temp) -> Add1/7
  [Cell_Current] -> Cell21/1(Cell_Current)
  [Cell_Current] -> Cell12/1(Cell_Current)
  [Cell_Current] -> Cell4/1(Cell_Current)
  Cell18/1(Cell_Voltage) -> Add/18
  Cell20/1(Cell_Voltage) -> Add/20
  Cell11/2(Cell_temp) -> Add1/11
  [Cell_Current] -> Cell2/1(Cell_Current)
  Cell16/2(Cell_temp) -> Add1/16
  [Cell_Current] -> Cell15/1(Cell_Current)
  [Cell_Current] -> Cell6/1(Cell_Current)
  [Cell_Current] -> Cell13/1(Cell_Current)
  Cell2/2(Cell_temp) -> Add1/2
  Cell22/2(Cell_temp) -> Add1/22
  Cell9/1(Cell_Voltage) -> Add/9
  Cell7/1(Cell_Voltage) -> Add/7
  [Cell_Current] -> Cell9/1(Cell_Current)
  Cell14/2(Cell_temp) -> Add1/14
  Cell17/1(Cell_Voltage) -> Add/17
  Cell10/2(Cell_temp) -> Add1/10
  [Cell_Current] -> Cell16/1(Cell_Current)
  Cell8/1(Cell_Voltage) -> Add/8
  Cell21/1(Cell_Voltage) -> Add/21
  Cell12/2(Cell_temp) -> Add1/12
  Cell22/1(Cell_Voltage) -> Add/22
  [Cell_Current] -> Cell20/1(Cell_Current)
  [Cell_Current] -> Cell17/1(Cell_Current)
  Cell10/1(Cell_Voltage) -> Add/10
  Cell18/2(Cell_temp) -> Add1/18
  Cell14/1(Cell_Voltage) -> Add/14
  Cell16/1(Cell_Voltage) -> Add/16
  [Cell_Current] -> Cell3/1(Cell_Current)
  Cell12/1(Cell_Voltage) -> Add/12
  Cell20/2(Cell_temp) -> Add1/20
  Cell1/1(Cell_Voltage) -> Add/1
  [Cell_Current] -> Cell19/1(Cell_Current)
  Cell3/1(Cell_Voltage) -> Add/3
  [Cell_Current] -> Cell22/1(Cell_Current)
  [Cell_Current] -> Cell14/1(Cell_Current)
  Cell19/2(Cell_temp) -> Add1/19
  Cell6/2(Cell_temp) -> Add1/6
  Cell17/2(Cell_temp) -> Add1/17
  Cell15/2(Cell_temp) -> Add1/15
  Cell8/2(Cell_temp) -> Add1/8
  Cell3/2(Cell_temp) -> Add1/3
  Cell13/2(Cell_temp) -> Add1/13
  Add/1 -> SubModule_Voltage/1
  Cell4/2(Cell_temp) -> Add1/4
  Cell5/2(Cell_temp) -> Add1/5
  Cell1/2(Cell_temp) -> Add1/1
  Add1/1 -> Divide/1
  Constant/1 -> Divide/2
  Divide/1 -> SubModule_avg_temp/1

== system Final_Dual2/Battery1/Module1/SubModule_6 ==
  Module_Current : Inport
  Add : Sum  Inputs=++++++++++++++++++++++
  Add1 : Sum  Inputs=++++++++++++++++++++++
  Cell1 : Subsystem
  Cell10 : Subsystem
  Cell11 : Subsystem
  Cell12 : Subsystem
  Cell13 : Subsystem
  Cell14 : Subsystem
  Cell15 : Subsystem
  Cell16 : Subsystem
  Cell17 : Subsystem
  Cell18 : Subsystem
  Cell19 : Subsystem
  Cell2 : Subsystem
  Cell20 : Subsystem
  Cell21 : Subsystem
  Cell22 : Subsystem
  Cell3 : Subsystem
  Cell4 : Subsystem
  Cell5 : Subsystem
  Cell6 : Subsystem
  Cell7 : Subsystem
  Cell8 : Subsystem
  Cell9 : Subsystem
  Constant : Constant  Value=22
  Divide : Product  Inputs=*/
  SubModule_Voltage : Outport
  SubModule_avg_temp : Outport  Port=2
  wires:
  Divide/1 -> SubModule_avg_temp/1
  Constant/1 -> Divide/2
  Add1/1 -> Divide/1
  Cell1/2(Cell_temp) -> Add1/1
  Cell5/2(Cell_temp) -> Add1/5
  Cell4/2(Cell_temp) -> Add1/4
  Add/1 -> SubModule_Voltage/1
  Cell13/2(Cell_temp) -> Add1/13
  Cell3/2(Cell_temp) -> Add1/3
  Cell8/2(Cell_temp) -> Add1/8
  Cell15/2(Cell_temp) -> Add1/15
  Cell17/2(Cell_temp) -> Add1/17
  Cell6/2(Cell_temp) -> Add1/6
  Cell19/2(Cell_temp) -> Add1/19
  [Cell_Current] -> Cell14/1(Cell_Current)
  [Cell_Current] -> Cell22/1(Cell_Current)
  Cell3/1(Cell_Voltage) -> Add/3
  [Cell_Current] -> Cell19/1(Cell_Current)
  Cell1/1(Cell_Voltage) -> Add/1
  Cell20/2(Cell_temp) -> Add1/20
  Cell12/1(Cell_Voltage) -> Add/12
  [Cell_Current] -> Cell3/1(Cell_Current)
  Cell16/1(Cell_Voltage) -> Add/16
  Cell14/1(Cell_Voltage) -> Add/14
  Cell18/2(Cell_temp) -> Add1/18
  Cell10/1(Cell_Voltage) -> Add/10
  [Cell_Current] -> Cell17/1(Cell_Current)
  [Cell_Current] -> Cell20/1(Cell_Current)
  Cell22/1(Cell_Voltage) -> Add/22
  Cell12/2(Cell_temp) -> Add1/12
  Cell21/1(Cell_Voltage) -> Add/21
  Cell8/1(Cell_Voltage) -> Add/8
  [Cell_Current] -> Cell16/1(Cell_Current)
  Cell10/2(Cell_temp) -> Add1/10
  Cell17/1(Cell_Voltage) -> Add/17
  Cell14/2(Cell_temp) -> Add1/14
  [Cell_Current] -> Cell9/1(Cell_Current)
  Cell7/1(Cell_Voltage) -> Add/7
  Cell9/1(Cell_Voltage) -> Add/9
  Cell22/2(Cell_temp) -> Add1/22
  Cell2/2(Cell_temp) -> Add1/2
  [Cell_Current] -> Cell13/1(Cell_Current)
  [Cell_Current] -> Cell6/1(Cell_Current)
  [Cell_Current] -> Cell15/1(Cell_Current)
  Cell16/2(Cell_temp) -> Add1/16
  [Cell_Current] -> Cell2/1(Cell_Current)
  Cell11/2(Cell_temp) -> Add1/11
  Cell20/1(Cell_Voltage) -> Add/20
  Cell18/1(Cell_Voltage) -> Add/18
  [Cell_Current] -> Cell4/1(Cell_Current)
  [Cell_Current] -> Cell12/1(Cell_Current)
  [Cell_Current] -> Cell21/1(Cell_Current)
  Cell7/2(Cell_temp) -> Add1/7
  [Cell_Current] -> Cell18/1(Cell_Current)
  Cell11/1(Cell_Voltage) -> Add/11
  Cell6/1(Cell_Voltage) -> Add/6
  [Cell_Current] -> Cell11/1(Cell_Current)
  [Cell_Current] -> Cell5/1(Cell_Current)
  Cell19/1(Cell_Voltage) -> Add/19
  Cell2/1(Cell_Voltage) -> Add/2
  [Cell_Current] -> Cell1/1(Cell_Current)
  Cell5/1(Cell_Voltage) -> Add/5
  Cell21/2(Cell_temp) -> Add1/21
  [Cell_Current] -> Cell10/1(Cell_Current)
  [Cell_Current] -> Cell7/1(Cell_Current)
  Cell15/1(Cell_Voltage) -> Add/15
  Module_Current/1 -> [Cell_Current]
  Cell4/1(Cell_Voltage) -> Add/4
  Cell13/1(Cell_Voltage) -> Add/13
  [Cell_Current] -> Cell8/1(Cell_Current)
  Cell9/2(Cell_temp) -> Add1/9

== system Final_Dual2/Battery1/Module1/SubModule_7 ==
  Module_Current : Inport
  Add : Sum  Inputs=++++++++++++++++++++++
  Add1 : Sum  Inputs=++++++++++++++++++++++
  Cell1 : Subsystem
  Cell10 : Subsystem
  Cell11 : Subsystem
  Cell12 : Subsystem
  Cell13 : Subsystem
  Cell14 : Subsystem
  Cell15 : Subsystem
  Cell16 : Subsystem
  Cell17 : Subsystem
  Cell18 : Subsystem
  Cell19 : Subsystem
  Cell2 : Subsystem
  Cell20 : Subsystem
  Cell21 : Subsystem
  Cell22 : Subsystem
  Cell3 : Subsystem
  Cell4 : Subsystem
  Cell5 : Subsystem
  Cell6 : Subsystem
  Cell7 : Subsystem
  Cell8 : Subsystem
  Cell9 : Subsystem
  Constant : Constant  Value=22
  Divide : Product  Inputs=*/
  SubModule_Voltage : Outport
  SubModule_avg_temp : Outport  Port=2
  wires:
  Divide/1 -> SubModule_avg_temp/1
  Constant/1 -> Divide/2
  Add1/1 -> Divide/1
  Cell1/2(Cell_temp) -> Add1/1
  Cell5/2(Cell_temp) -> Add1/5
  Cell4/2(Cell_temp) -> Add1/4
  Add/1 -> SubModule_Voltage/1
  Cell13/2(Cell_temp) -> Add1/13
  Cell3/2(Cell_temp) -> Add1/3
  Cell8/2(Cell_temp) -> Add1/8
  Cell15/2(Cell_temp) -> Add1/15
  Cell17/2(Cell_temp) -> Add1/17
  Cell6/2(Cell_temp) -> Add1/6
  Cell19/2(Cell_temp) -> Add1/19
  [Cell_Current] -> Cell14/1(Cell_Current)
  [Cell_Current] -> Cell22/1(Cell_Current)
  Cell3/1(Cell_Voltage) -> Add/3
  [Cell_Current] -> Cell19/1(Cell_Current)
  Cell1/1(Cell_Voltage) -> Add/1
  Cell20/2(Cell_temp) -> Add1/20
  Cell12/1(Cell_Voltage) -> Add/12
  [Cell_Current] -> Cell3/1(Cell_Current)
  Cell16/1(Cell_Voltage) -> Add/16
  Cell14/1(Cell_Voltage) -> Add/14
  Cell18/2(Cell_temp) -> Add1/18
  Cell10/1(Cell_Voltage) -> Add/10
  [Cell_Current] -> Cell17/1(Cell_Current)
  [Cell_Current] -> Cell20/1(Cell_Current)
  Cell22/1(Cell_Voltage) -> Add/22
  Cell12/2(Cell_temp) -> Add1/12
  Cell21/1(Cell_Voltage) -> Add/21
  Cell8/1(Cell_Voltage) -> Add/8
  [Cell_Current] -> Cell16/1(Cell_Current)
  Cell10/2(Cell_temp) -> Add1/10
  Cell17/1(Cell_Voltage) -> Add/17
  Cell14/2(Cell_temp) -> Add1/14
  [Cell_Current] -> Cell9/1(Cell_Current)
  Cell7/1(Cell_Voltage) -> Add/7
  Cell9/1(Cell_Voltage) -> Add/9
  Cell22/2(Cell_temp) -> Add1/22
  Cell2/2(Cell_temp) -> Add1/2
  [Cell_Current] -> Cell13/1(Cell_Current)
  [Cell_Current] -> Cell6/1(Cell_Current)
  [Cell_Current] -> Cell15/1(Cell_Current)
  Cell16/2(Cell_temp) -> Add1/16
  [Cell_Current] -> Cell2/1(Cell_Current)
  Cell11/2(Cell_temp) -> Add1/11
  Cell20/1(Cell_Voltage) -> Add/20
  Cell18/1(Cell_Voltage) -> Add/18
  [Cell_Current] -> Cell4/1(Cell_Current)
  [Cell_Current] -> Cell12/1(Cell_Current)
  [Cell_Current] -> Cell21/1(Cell_Current)
  Cell7/2(Cell_temp) -> Add1/7
  [Cell_Current] -> Cell18/1(Cell_Current)
  Cell11/1(Cell_Voltage) -> Add/11
  Cell6/1(Cell_Voltage) -> Add/6
  [Cell_Current] -> Cell11/1(Cell_Current)
  [Cell_Current] -> Cell5/1(Cell_Current)
  Cell19/1(Cell_Voltage) -> Add/19
  Cell2/1(Cell_Voltage) -> Add/2
  [Cell_Current] -> Cell1/1(Cell_Current)
  Cell5/1(Cell_Voltage) -> Add/5
  Cell21/2(Cell_temp) -> Add1/21
  [Cell_Current] -> Cell10/1(Cell_Current)
  [Cell_Current] -> Cell7/1(Cell_Current)
  Cell15/1(Cell_Voltage) -> Add/15
  Module_Current/1 -> [Cell_Current]
  Cell4/1(Cell_Voltage) -> Add/4
  Cell13/1(Cell_Voltage) -> Add/13
  [Cell_Current] -> Cell8/1(Cell_Current)
  Cell9/2(Cell_temp) -> Add1/9
